simulink model "Q3_M1"  (R2024b)
settings: Solver=VariableStepAuto  StartTime=0.0  StopTime=10.0  RelTol=1e-3
settings Model: Creator=chall  LastModifiedBy=chall

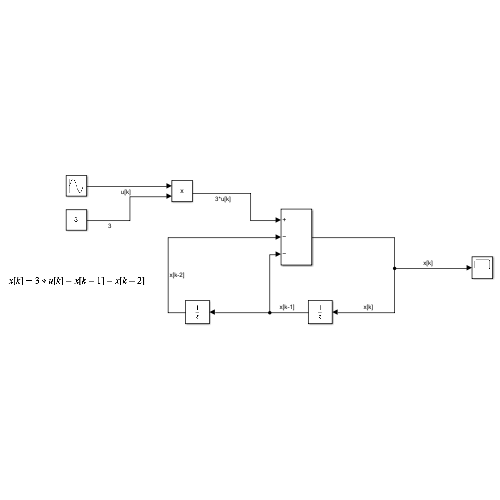
[thumbnail: Simulink's stored preview of the top-level diagram]
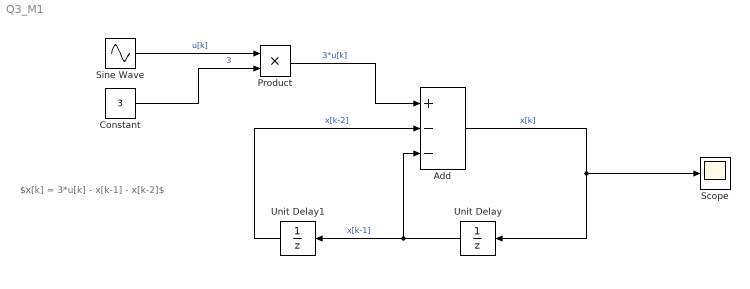
== system Q3_M1 ==
  note: $x[k] = 3*u[k] - x[k-1] - x[k-2]$
  Add : Sum  Inputs=+--
  Constant : Constant  Value=3
  Product : Product
  Scope : Scope
  Sine Wave : Sin  SampleTime=0
  Unit Delay : UnitDelay  SampleTime=-1  HasFrameUpgradeWarning=on
  Unit Delay1 : UnitDelay  SampleTime=-1  HasFrameUpgradeWarning=on
  wires:
  Add/1 -> Unit Delay/1, Scope/1  "x[k]"
  Unit Delay/1 -> Unit Delay1/1, Add/3  "x[k-1]"
  Unit Delay1/1 -> Add/2  "x[k-2]"
  Sine Wave/1 -> Product/1  "u[k]"
  Constant/1 -> Product/2  "3"
  Product/1 -> Add/1  "3*u[k]"
